simulink model "ex_5"  (R2016a)
settings: Solver=VariableStepAuto  StartTime=0.0  StopTime=10.0  RelTol=1e-3
settings Model: Creator=Linstar  LastModifiedBy=Linstar

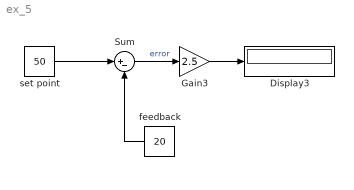
== system ex_5 ==
  Display3 : Display
  Gain3 : Gain  Gain=2.5
  Sum : Sum  Inputs=|+-
  feedback : Constant  Value=20
  set point : Constant  Value=50
  wires:
  set point/1 -> Sum/1
  Sum/1 -> Gain3/1  "error"
  feedback/1 -> Sum/2
  Gain3/1 -> Display3/1
